simulink model "proyectoventilador"  (R2020a)
settings: Solver=VariableStepAuto  StartTime=0.0  StopTime=2.5  FixedStep=0.001  RelTol=1e-3
values from neighbouring files (symbols this model uses):
  A = []    [caso.m]    (also in casom.m; simulacion.m = [[0 1]; [-(N1/N2)^2 * ka/J -(D+ kt*kb/R)/J]])
  AA = [[0 1 0 0]; [-(N1/N2)^2 * ka/J -(D+ kt*kb/R)/J 0 0]; [0 0 0 1]; [0 0 0 -(D1/Jm + kt/R * 1/Jm)]]    [simulacion.m]
  B = 0.01    [dinamica.m]    (also in simulacion.m = [0 ; kt/(R * J)])
  BB = [0 ; kt/(R * Jm); 0; kt/(R * Jm)]    [simulacion.m]
  CC = [[1 0 0 0]; [0 1 0 0]]    [simulacion.m]
  K1 = lqi (sys_ol, Q, R)    [simulacion.m]
  Ki = [K1(3) K1(3)]    [simulacion.m]
libraries: simulink x4
settings Model: Creator=charlie772  LastModifiedBy=root

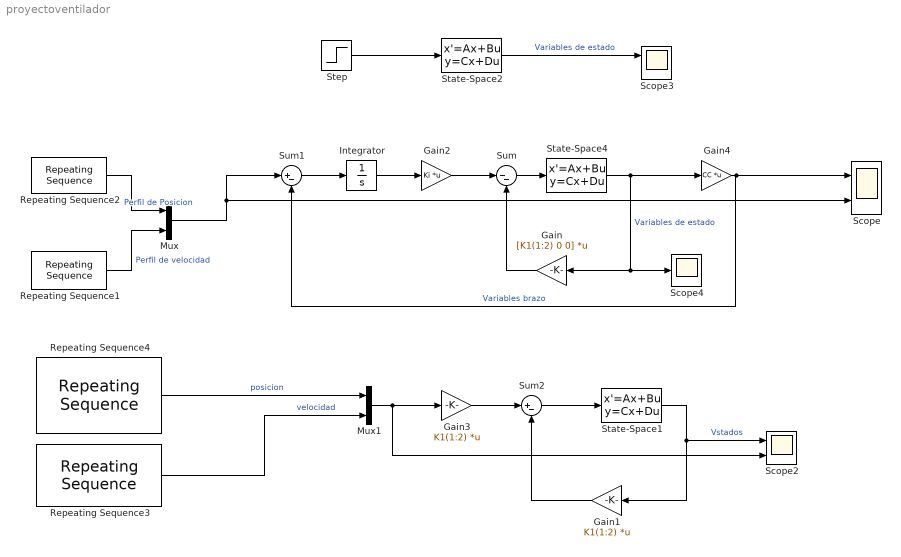
== system proyectoventilador ==
  Gain : Gain  Gain=[K1(1:2) 0 0]  Multiplication=Matrix(K*u) (u vector)
  Gain1 : Gain  Gain=K1(1:2)  Multiplication=Matrix(K*u) (u vector)
  Gain2 : Gain  Gain=Ki  Multiplication=Matrix(K*u) (u vector)
  Gain3 : Gain  Gain=K1(1:2)  Multiplication=Matrix(K*u) (u vector)
  Gain4 : Gain  Gain=CC  Multiplication=Matrix(K*u) (u vector)
  Integrator : Integrator
  Mux : Mux  Inputs=2
  Mux1 : Mux  Inputs=2
  Repeating Sequence1 : simulink/Sources/Repeating Sequence  rep_seq_t=t  rep_seq_y=vel_ajustado
  Repeating Sequence2 : simulink/Sources/Repeating Sequence  rep_seq_t=t  rep_seq_y=pos_norm
  Repeating Sequence3 : simulink/Sources/Repeating Sequence  rep_seq_t=t  rep_seq_y=vel_ajustado
  Repeating Sequence4 : simulink/Sources/Repeating Sequence  rep_seq_t=t  rep_seq_y=pos_norm
  Scope : Scope  NumInputPorts=2
  Scope2 : Scope  NumInputPorts=2
  Scope3 : Scope  NumInputPorts=2
  Scope4 : Scope
  State-Space1 : StateSpace  A=A  B=B  C=eye(2)  D=[0;0]  InitialCondition=0
  State-Space2 : StateSpace  A=AA  B=BB  C=eye(4)  D=[0;0;0;0]  InitialCondition=0
  State-Space4 : StateSpace  A=AA  B=BB  C=eye(4)  D=[0;0;0;0]  InitialCondition=0
  Step : Step  Time=0  SampleTime=0
  Sum : Sum  Inputs=|--
  Sum1 : Sum  Inputs=|+-
  Sum2 : Sum  Inputs=|+-
  wires:
  Gain/1 -> Sum/2
  Sum/1 -> State-Space4/1
  Repeating Sequence2/1 -> Mux/1  "Perfil de Posicion"
  Repeating Sequence1/1 -> Mux/2  "Perfil de velocidad"
  Mux/1 -> Scope/2, Sum1/1
  Integrator/1 -> Gain2/1
  Gain2/1 -> Sum/1
  Sum1/1 -> Integrator/1
  Gain3/1 -> Sum2/1
  State-Space1/1 -> Gain1/1, Scope2/1  "Vstados"
  Gain1/1 -> Sum2/2
  Sum2/1 -> State-Space1/1
  Step/1 -> State-Space2/1
  State-Space2/1 -> Scope3/1  "Variables de estado"
  Gain4/1 -> Sum1/2, Scope/1  "Variables brazo"
  State-Space4/1 -> Gain4/1, Scope4/1, Gain/1  "Variables de estado"
  Mux1/1 -> Scope2/2, Gain3/1
  Repeating Sequence4/1 -> Mux1/1  "posicion"
  Repeating Sequence3/1 -> Mux1/2  "velocidad"
